simulink model "SMC4PIBC"  (R2024a)
settings: Solver=ode1  StartTime=0.0  StopTime=10  RelTol=1e-3
values from neighbouring files (symbols this model uses):
  C = 100e-6    (= 0.0001)    [converterParametersfor4phase.m]
  r_load = 5    [converterParametersfor4phase.m]
  V_fc = 14.4    [converterParametersfor4phase.m]
undefined symbols (not defined in the file or in its folder): plecs
libraries: eePwmGenerator x4
settings Model: Creator=qaromose  LastModifiedBy=QUDUS
settings DebuggingCC: UnconnectedInputMsg=warning  UnconnectedOutputMsg=warning  UnconnectedLineMsg=warning
settings ModelReferenceCC: EnableRefExpFcnMdlSchedulingChecks=on
settings RTWCC: GPUComputeCapability=3.5  DLArmComputeVersion=19.05

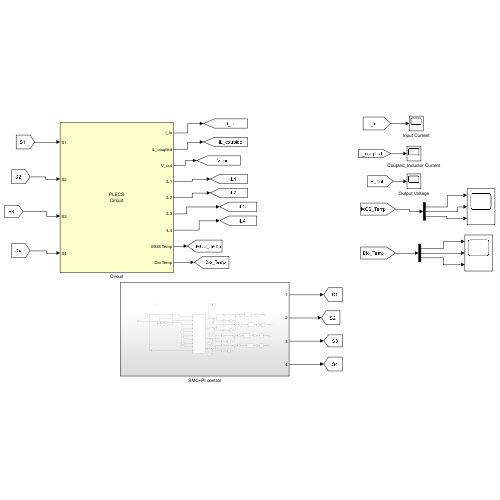
[thumbnail: Simulink's stored preview of the top-level diagram]
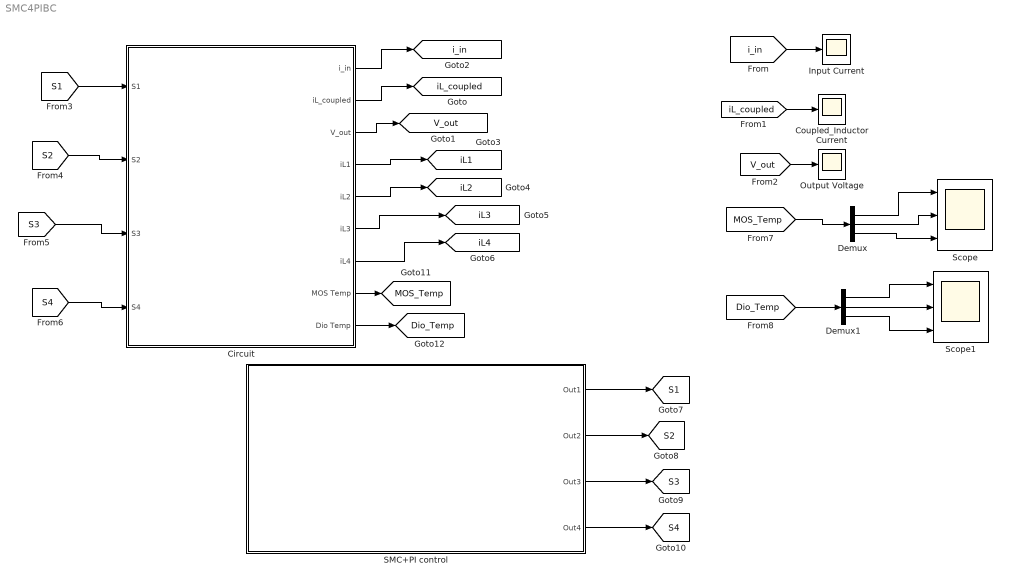
== system SMC4PIBC ==
  Circuit : Subsystem  LoadFcn=plecs('sl', 200);  InitFcn=plecs('sl', 214);  StartFcn=plecs('sl', 208);  StopFcn=plecs('sl', 209);  mask(PlecsCircuit){PLECSData=<binary blob, 18932 chars, not shown>}
      mask prompts: PLECSData "PLECS Data (Do not delete or modify!)"
      mask init:
      | % PLACE CUSTOM INITIALIZATIONS ABOVE
      | % DO NOT REMOVE
      | plecs('sl', 215);
      | % DO NOT REMOVE
      settings: CopyFcn=plecs('sl', 203);  DeleteFcn=plecs('sl', 205);  UndoDeleteFcn=plecs('sl', 206);  PreSaveFcn=plecs('sl', 211);  PostSaveFcn=plecs('sl', 201);  NameChangeFcn=plecs('sl', 210);  DestroyFcn=plecs('sl', 207);  PreCopyFcn=plecs('sl', 216);  OpenFcn=plecs('sl', 202);  ErrorFcn=plerrorfcn
      mask Help: eval('plecs(''help'', ''qthelp:///creatingacircuit.html'')')
      mask Display: disp('PLECS\nCircuit')
  Coupled_Inductor Current : Scope
  Demux : Demux  Outputs=3
  Demux1 : Demux  Outputs=3
  Input Current : Scope
  Output Voltage : Scope
  SMC+PI control : Subsystem
  Scope : Scope  NumInputPorts=3
  Scope1 : Scope  NumInputPorts=3
  tag scope: Dio_Temp=global, MOS_Temp=global, S1=global, S2=global, S3=global, S4=global, V_out=global, iL1=global, iL2=global, iL3=global, iL4=global, iL_coupled=global, i_in=global
  wires:
  [iL_coupled] -> Coupled_Inductor Current/1
  [V_out] -> Output Voltage/1
  Circuit/1(i_in) -> [i_in]
  Circuit/2(iL_coupled) -> [iL_coupled]
  Circuit/3(V_out) -> [V_out]
  [i_in] -> Input Current/1
  Circuit/4(iL1) -> [iL1]
  Circuit/5(iL2) -> [iL2]
  Circuit/6(iL3) -> [iL3]
  Circuit/7(iL4) -> [iL4]
  SMC+PI control/1(Out1) -> [S1]
  SMC+PI control/4(Out4) -> [S4]
  SMC+PI control/3(Out3) -> [S3]
  SMC+PI control/2(Out2) -> [S2]
  [S1] -> Circuit/1(S1)
  [S2] -> Circuit/2(S2)
  [S3] -> Circuit/3(S3)
  [S4] -> Circuit/4(S4)
  Circuit/8(MOS Temp) -> [MOS_Temp]
  Circuit/9(Dio Temp) -> [Dio_Temp]
  [MOS_Temp] -> Demux/1
  [Dio_Temp] -> Demux1/1
  Demux/1 -> Scope/1
  Demux/2 -> Scope/2
  Demux/3 -> Scope/3
  Demux1/1 -> Scope1/1
  Demux1/2 -> Scope1/2
  Demux1/3 -> Scope1/3

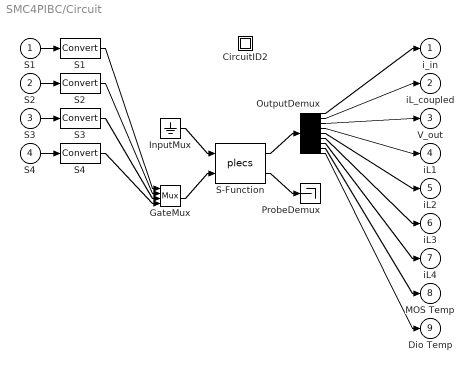
== system SMC4PIBC/Circuit ==
  S1 : Inport  PortDimensions=1
  S2 : Inport  Port=2  PortDimensions=1
  S3 : Inport  Port=3  PortDimensions=1
  S4 : Inport  Port=4  PortDimensions=1
  " CircuitID2 " : Subsystem
  " GateMux " : Mux  Inputs=[ 1 1 1 1 ]
  " InputMux " : Ground
  " OutputDemux " : Demux  Outputs=[ 1 4 1 1 1 1 1 3 3 ]
  " ProbeDemux " : Terminator
  " S-Function " : S-Function  FunctionName=plecs  SFunctionDeploymentMode=off  EnableBusSupport=off
  " S1 " : DataTypeConversion
  " S2 " : DataTypeConversion
  " S3 " : DataTypeConversion
  " S4 " : DataTypeConversion
  i_in : Outport  PortDimensions=1
  iL_coupled : Outport  Port=2  PortDimensions=4
  V_out : Outport  Port=3  PortDimensions=1
  iL1 : Outport  Port=4  PortDimensions=1
  iL2 : Outport  Port=5  PortDimensions=1
  iL3 : Outport  Port=6  PortDimensions=1
  iL4 : Outport  Port=7  PortDimensions=1
  MOS Temp : Outport  Port=8  PortDimensions=3
  Dio Temp : Outport  Port=9  PortDimensions=3
  wires:
  " InputMux "/1 -> " S-Function "/1
  " GateMux "/1 -> " S-Function "/2
  " S-Function "/1 -> " OutputDemux "/1
  " S-Function "/2 -> " ProbeDemux "/1
  S1/1 -> " S1 "/1
  " S1 "/1 -> " GateMux "/1
  S2/1 -> " S2 "/1
  " S2 "/1 -> " GateMux "/2
  S3/1 -> " S3 "/1
  " S3 "/1 -> " GateMux "/3
  S4/1 -> " S4 "/1
  " S4 "/1 -> " GateMux "/4
  " OutputDemux "/1 -> i_in/1
  " OutputDemux "/2 -> iL_coupled/1
  " OutputDemux "/3 -> V_out/1
  " OutputDemux "/4 -> iL1/1
  " OutputDemux "/5 -> iL2/1
  " OutputDemux "/6 -> iL3/1
  " OutputDemux "/7 -> iL4/1
  " OutputDemux "/8 -> MOS Temp/1
  " OutputDemux "/9 -> Dio Temp/1

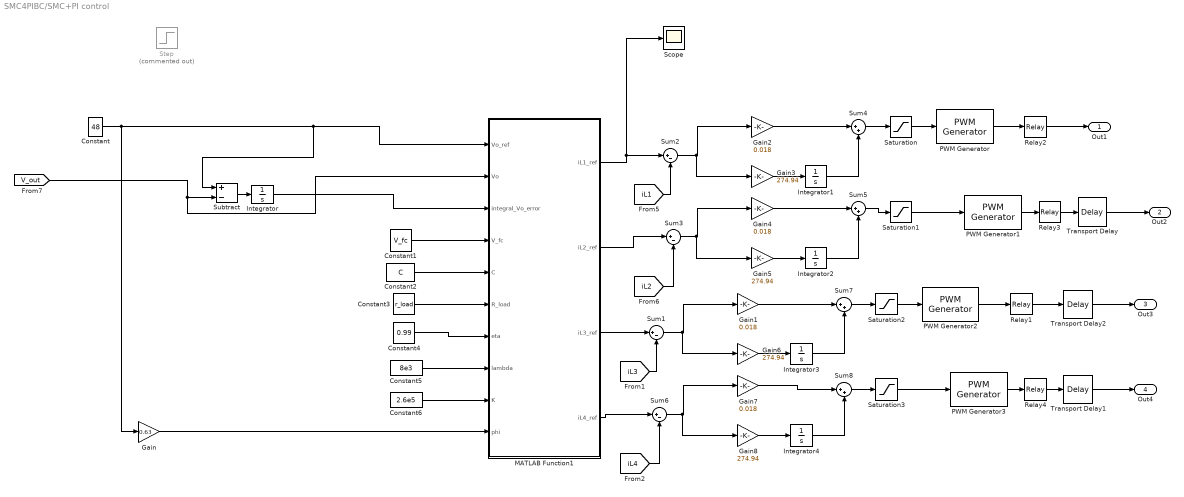
== system SMC4PIBC/SMC+PI control ==
  Constant : Constant  Value=48
  Constant1 : Constant  Value=V_fc
  Constant2 : Constant  Value=C
  Constant3 : Constant  Value=r_load
  Constant4 : Constant  Value=0.99
  Constant5 : Constant  Value=8e3
  Constant6 : Constant  Value=2.6e5
  Gain : Gain  Gain=0.63
  Gain{1..2,4,7} (4 alike) : Gain  Gain=0.018
  Gain{3,5..6,8} (4 alike) : Gain  Gain=274.94
  Integrator{,1..4} (5 alike) : Integrator
  MATLAB Function1 : MATLAB Function  TreatAsAtomicUnit=on
  PWM Generator{,1..3} (4 alike) : eePwmGenerator/PWM Generator  CarrCount=Up  Tper=2e-5  Tdelay=0  Ts=0
  Relay{1..4} (4 alike) : Relay
  Saturation{,1..3} (4 alike) : Saturate  UpperLimit=0.97  LowerLimit=0.1
  Scope : Scope
  Step : Step  Commented=on  Time=5  Before=48  After=40  SampleTime=0
  Subtract : Sum  Inputs=+-
  Sum{1..3,6} (4 alike) : Sum  Inputs=|+-
  Sum{4..5,7..8} (4 alike) : Sum  Inputs=|++
  Transport Delay : TransportDelay  DelayTime=5e-6
  Transport Delay1 : TransportDelay  DelayTime=1.5e-5
  Transport Delay2 : TransportDelay  DelayTime=1e-5
  Out1 : Outport
  Out2 : Outport  Port=2
  Out3 : Outport  Port=3
  Out4 : Outport  Port=4
  wires:
  Relay2/1 -> Out1/1
  Relay3/1 -> Transport Delay/1
  Sum2/1 -> Gain3/1, Gain2/1
  [V_out] -> Subtract/2, MATLAB Function1/2(Vo)
  Saturation/1 -> PWM Generator/1
  [iL1] -> Sum2/2
  Subtract/1 -> Integrator/1
  Transport Delay/1 -> Out2/1
  Sum3/1 -> Gain5/1, Gain4/1
  MATLAB Function1/1(iL1_ref) -> Scope/1, Sum2/1
  MATLAB Function1/2(iL2_ref) -> Sum3/1
  PWM Generator/1 -> Relay2/1
  Gain4/1 -> Sum5/1
  Sum4/1 -> Saturation/1
  Gain5/1 -> Integrator2/1
  Integrator2/1 -> Sum5/2
  Gain3/1 -> Integrator1/1
  PWM Generator1/1 -> Relay3/1
  Integrator1/1 -> Sum4/2
  Integrator/1 -> MATLAB Function1/3(integral_Vo_error)
  Gain2/1 -> Sum4/1
  Saturation1/1 -> PWM Generator1/1
  Sum5/1 -> Saturation1/1
  [iL2] -> Sum3/2
  Constant2/1 -> MATLAB Function1/5(C)
  Constant3/1 -> MATLAB Function1/6(R_load)
  Constant4/1 -> MATLAB Function1/7(eta)
  Constant5/1 -> MATLAB Function1/8(lambda)
  Constant6/1 -> MATLAB Function1/9(K)
  Gain/1 -> MATLAB Function1/10(phi)
  Constant1/1 -> MATLAB Function1/4(V_fc)
  MATLAB Function1/4(iL4_ref) -> Sum6/1
  PWM Generator2/1 -> Relay1/1
  Sum1/1 -> Gain6/1, Gain1/1
  [iL4] -> Sum6/2
  Saturation3/1 -> PWM Generator3/1
  Gain1/1 -> Sum7/1
  Saturation2/1 -> PWM Generator2/1
  Gain7/1 -> Sum8/1
  Integrator3/1 -> Sum7/2
  Relay1/1 -> Transport Delay2/1
  Transport Delay1/1 -> Out4/1
  Gain6/1 -> Integrator3/1
  MATLAB Function1/3(iL3_ref) -> Sum1/1
  Gain8/1 -> Integrator4/1
  PWM Generator3/1 -> Relay4/1
  [iL3] -> Sum1/2
  Sum8/1 -> Saturation3/1
  Relay4/1 -> Transport Delay1/1
  Sum7/1 -> Saturation2/1
  Integrator4/1 -> Sum8/2
  Sum6/1 -> Gain8/1, Gain7/1
  Transport Delay2/1 -> Out3/1
  Constant/1 -> Subtract/1, MATLAB Function1/1(Vo_ref), Gain/1

== system SMC4PIBC/Circuit/ CircuitID2  ==

== matlab function SMC4PIBC/SMC+PI control/MATLAB Function1 ==
  data: Vo_ref input; Vo input; integral_Vo_error input; iL1_ref output; iL2_ref output; V_fc input; C input; R_load input; eta input; lambda input; K input; phi input; iL3_ref output; iL4_ref output
function [iL1_ref, iL2_ref, iL3_ref, iL4_ref] = Outer_SMC(Vo_ref, Vo, integral_Vo_error, V_fc, C, R_load, eta, lambda, K, phi)
    %% System Parameters (Optimized for ±0.5V Error)
%     V_fc = 14.4;          % Input voltage [V] (measured under load)
%     C = 100e-6;          % Output capacitance [F] 
%     R_load = 5;          % Load resistance [Ω] (48V/500W = 4.608Ω, adjust if needed)
%     eta = 0.97;          % desired efficiency (compensate for losses at higher Vo)
%     lambda = 2500;       % Aggressive integral gain (eliminate steady-state error)
%     K = 600;             % High robustness gain (dominate uncertainties)
%     phi = 0.5 * Vo_ref;% Adaptive boundary layer (0.5% of Vo_ref)
    
    %% Voltage error (Vo_ref - Vo)
    e_V = Vo_ref - Vo;
    
    %% Sliding surface
    S = e_V + lambda * integral_Vo_error;
    
    %% Adaptive boundary layer saturation
    if abs(S) <= phi
        sat_term = S / phi;   % Linear region
    else
        sat_term = sign(S);   % Reaching mode
    end
    
    %% Feedforward term (with efficiency compensation)
    iL_ref_eq = (Vo_ref^2) / (V_fc * R_load * eta);  % Critical adjustment
    
    %% Feedback term (scaled for precision)
    robustness_term = (C / V_fc) * (lambda * e_V + K * sat_term); 
    
    %% Total current reference (remove clamp or set hardware-safe limit)
    iL_ref_total = iL_ref_eq + robustness_term;
    % iL_ref_total = max(min(iL_ref_total, 100), 0);  % Example: 100A limit
    
    %% Split equally for 4-phase IBC
    iL1_ref = iL_ref_total / 4;  
    iL2_ref = iL_ref_total / 4;
    iL3_ref = iL_ref_total / 4;  
    iL4_ref = iL_ref_total / 4;
end
